simulink model "lab2_sim"  (R2020b)
settings: Solver=VariableStepAuto  StartTime=0.0  StopTime=50  RelTol=1e-3
settings Model: Creator=student  LastModifiedBy=student

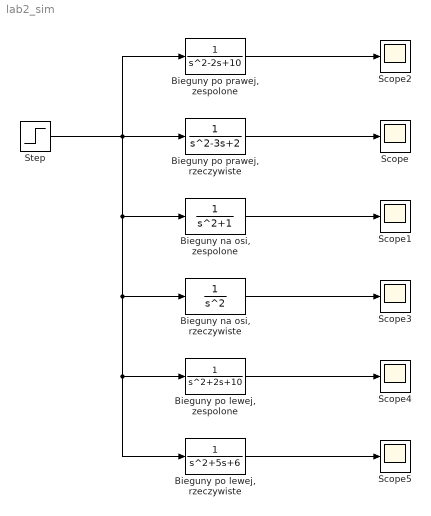
== system lab2_sim ==
  "Bieguny na osi, rzeczywiste" : TransferFcn  Denominator=[1 0 0]
  "Bieguny na osi, zespolone" : TransferFcn  Denominator=[1 0 1]
  "Bieguny po lewej, rzeczywiste" : TransferFcn  Denominator=[1 5 6]
  "Bieguny po lewej, zespolone" : TransferFcn  Denominator=[1 2 10]
  "Bieguny po prawej, rzeczywiste" : TransferFcn  Denominator=[1 -3 2]
  "Bieguny po prawej, zespolone" : TransferFcn  Denominator=[1 -2 10]
  Scope{,1..5} (6 alike) : Scope
  Step : Step  SampleTime=0
  wires:
  "Bieguny po prawej, rzeczywiste"/1 -> Scope/1
  "Bieguny na osi, zespolone"/1 -> Scope1/1
  "Bieguny po prawej, zespolone"/1 -> Scope2/1
  Step/1 -> "Bieguny po lewej, rzeczywiste"/1, "Bieguny po lewej, zespolone"/1, "Bieguny na osi, rzeczywiste"/1, "Bieguny na osi, zespolone"/1, "Bieguny po prawej, zespolone"/1, "Bieguny po prawej, rzeczywiste"/1
  "Bieguny po lewej, rzeczywiste"/1 -> Scope5/1
  "Bieguny po lewej, zespolone"/1 -> Scope4/1
  "Bieguny na osi, rzeczywiste"/1 -> Scope3/1
